simulink model "controlador_PID"  (R2023b)
settings: Solver=VariableStepAuto  StartTime=0.0  StopTime=10.0  RelTol=1e-3
values from neighbouring files (symbols this model uses):
  b_a = J_eq*(2*zitta+1)*w_pos    (= 0.0395694444444)    [constantes.m]
  K_sa = J_eq*(2*zitta+1)*w_pos^2    (= 31.6555555556)    [constantes.m]    (also in test_polos_PID.m = J_eq*n*w_pos^2)
  K_sia = J_eq*w_pos^3    (= 10129.7777778)    [constantes.m]    (also in test_polos_PID.m = J_eq*w_pos^3)
settings Model: Creator=rodri  LastModifiedBy=rodri

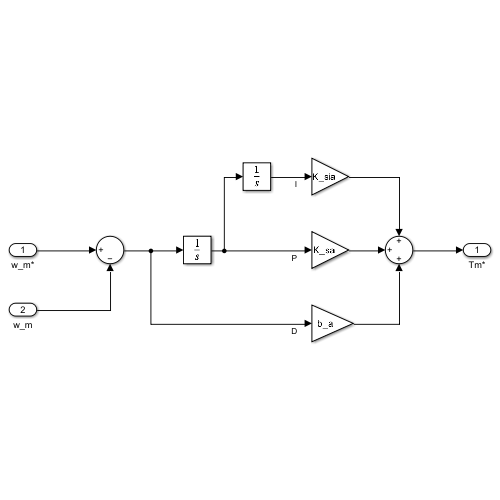
[thumbnail: Simulink's stored preview of the top-level diagram]
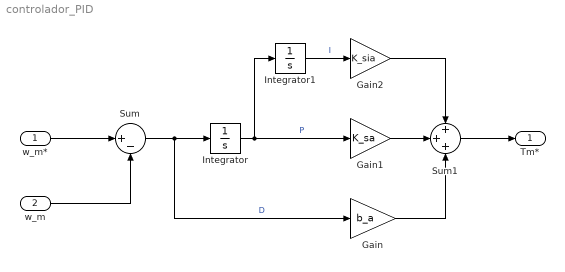
== system controlador_PID ==
  w_m* : Inport
  w_m : Inport  Port=2
  Gain : Gain  Gain=b_a
  Gain1 : Gain  Gain=K_sa
  Gain2 : Gain  Gain=K_sia
  Integrator : Integrator
  Integrator1 : Integrator
  Sum : Sum  Inputs=|+-
  Sum1 : Sum  Inputs=+++
  Tm* : Outport
  wires:
  w_m*/1 -> Sum/1
  w_m/1 -> Sum/2
  Sum/1 -> Gain/1, Integrator/1  "D"
  Integrator/1 -> Integrator1/1, Gain1/1  "P"
  Integrator1/1 -> Gain2/1  "I"
  Gain2/1 -> Sum1/1
  Gain1/1 -> Sum1/2
  Gain/1 -> Sum1/3
  Sum1/1 -> Tm*/1
